simulink model "SPI_inicjalizacja"  (R2019b)
settings: Solver=FixedStepAuto  StartTime=0.0  StopTime=inf  RelTol=1e-3  EnableMultiTasking=on
model workspace (MATLAB code in the model file):
  | function Vector_change = VEC(X,Y)
  | Vector_change = [X, Y]
libraries: simulink x1, raspberrypilib x1
settings Model: OrderedModelArguments=off  Creator=damia  LastModifiedBy=damia
settings SolverCC: PositivePriorityOrder=on  AutoInsertRateTranBlk=on
settings OptimizationCC: EnhancedBackFolding=on  PassReuseOutputArgsAs=Individual arguments  ZeroExternalMemoryAtStartup=off  ZeroInternalMemoryAtStartup=off  MaxStackSize=64  OptimizeBlockOrder=speed  DifferentSizesBufferReuse=on  OptimizationCustomize=off  EfficientTunableParamExpr=on
settings DebuggingCC: ParameterTunabilityLossMsg=error
settings HardwareCC: ProdBitPerPointer=32  ProdBitPerSizeT=32  ProdBitPerPtrDiffT=32  ProdLargestAtomicInteger=Long  ProdLargestAtomicFloat=Double  ProdWordSize=32  ProdLongLongMode=on  ProdHWDeviceType=ARM Compatible->ARM Cortex  UseEmbeddedCoderFeatures=off  UseSimulinkCoderFeatures=off
settings RTWCC: SystemTargetFile=ert.tlc  HardwareBoard=Raspberry Pi  TLCOptions="-aInlineSetEventsForThisBaseRateFcn=TLC_FALSE -aSuppressMultiTaskScheduler=TLC_FALSE  -aRateBasedStepFcn=0"  TemplateMakefile=ert_default_tmf  RTWVerbose=off  Toolchain=GNU GCC Raspberry Pi  BuildConfiguration=Faster Runs  IncludeHyperlinkInReport=on
settings CodeAppCC: ForceParamTrailComments=on  OperatorAnnotations=on  SimulinkDataObjDesc=on  SFDataObjDesc=on  InsertBlockDesc=on
settings ERTTargetCC: SupportNonInlinedSFcns=on  SupportVariableSizeSignals=on  ERTSrcFileBannerTemplate=codertarget_code_template.cgt  ERTHdrFileBannerTemplate=codertarget_code_template.cgt  ERTDataSrcFileTemplate=codertarget_code_template.cgt  ERTDataHdrFileTemplate=codertarget_code_template.cgt

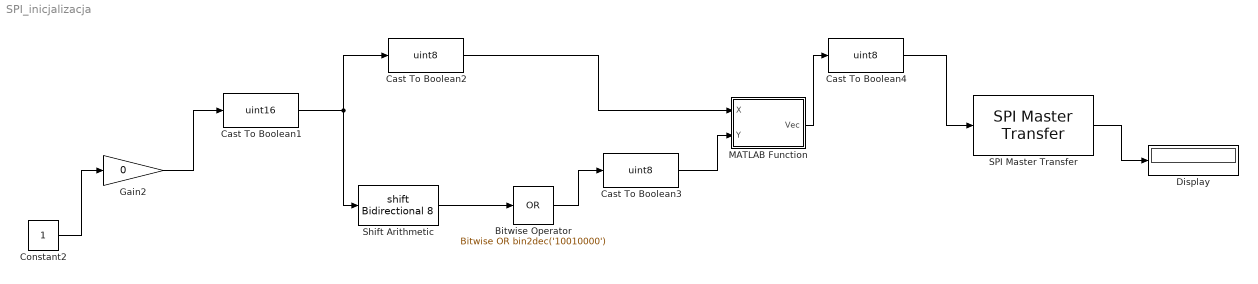
== system SPI_inicjalizacja ==
  Bitwise Operator : simulink/Logic and Bit Operations/Bitwise Operator  logicop=OR  UseBitMask=on  BitMask=bin2dec('10010000')  BitMaskRealWorld=Real World Value
  Cast To Boolean1 : DataTypeConversion  OutDataTypeStr=uint16
  Cast To Boolean2 : DataTypeConversion  OutDataTypeStr=uint8
  Cast To Boolean3 : DataTypeConversion  OutDataTypeStr=uint8
  Cast To Boolean4 : DataTypeConversion  OutDataTypeStr=uint8
  Constant2 : Constant
  Display : Display
  Gain2 : Gain  Gain=0
  MATLAB Function : MATLAB Function  TreatAsAtomicUnit=on
  SPI Master Transfer : raspberrypilib/SPI Master Transfer  Priority=1  BoardProperty=Pi 3 Model B  SPIModule=uint32(0)  Mode=Master  BusSpeed=1000000  Pin=SPI0_CE0  FirstBitToTransfer=Most significant bit (MSB)  ClockMode=0  BlockFunction=Transfer  RegisterAddress=0  OutputDataType=int8  OutputDataLength=1
      settings: SourceProductName=Simulink Support Package for Raspberry Pi Hardware  SourceProductBaseCode=RASPPI
  Shift Arithmetic : ArithShift  BitShiftNumber=8
  wires:
  Constant2/1 -> Gain2/1
  Gain2/1 -> Cast To Boolean1/1
  Cast To Boolean1/1 -> Cast To Boolean2/1, Shift Arithmetic/1
  Shift Arithmetic/1 -> Bitwise Operator/1
  Bitwise Operator/1 -> Cast To Boolean3/1
  Cast To Boolean2/1 -> MATLAB Function/1(X)
  Cast To Boolean3/1 -> MATLAB Function/2(Y)
  MATLAB Function/1(Vec) -> Cast To Boolean4/1
  SPI Master Transfer/1 -> Display/1
  Cast To Boolean4/1 -> SPI Master Transfer/1

== matlab function SPI_inicjalizacja/MATLAB Function ==
  data: X input; Vec output; Y input
function Vec = Vector(X, Y)

% myPI = raspi();
Vec = [Y X];
% mySPI = spidev(myPI,'CE0');
% out = writeRead(mySPI,[Vec]);
